simulink model "Robot_Control"  (Simulink 7.7)
settings: Solver=ode1  StartTime=0.0  StopTime=inf  FixedStep=0.002  RelTol=1e-3
values from neighbouring files (symbols this model uses):
  k = place(A,B,p)    [BalancePoles.m]
undefined symbols (not defined in the file or in its folder): HIL
libraries: quarc_library x4, simulink x1
settings Model: Creator=rcb4  LastModifiedBy=rcb4  SimulationMode=external  ExtModeTrigDuration=5000
settings SolverCC: PositivePriorityOrder=on
settings RTWCC: SystemTargetFile=quarc_win64.tlc  TemplateMakefile=quarc_default_tmf  Description=QUARC Win64 Target  ProcessScript=quarc_win64_make_rtw_hook
settings STFCustomTargetCC: TargetPreCompLibLocation=C:\PROGRA~3\QUARC\lib\2011a\win64\release  FunctionExecutionProfile=off  GeneratePreprocessorConditionals=Disable all  SystemTargetFile=quarc_win64.tlc
settings GRTTargetCC: TargetPreCompLibLocation=C:\PROGRA~3\QUARC\lib\2011a\win64\release  ParMdlRefBuildCompliant=off  CompOptLevelCompliant=off  MatFileLogging=off  ExtMode=on  ExtModeMexFile=quarc_comm

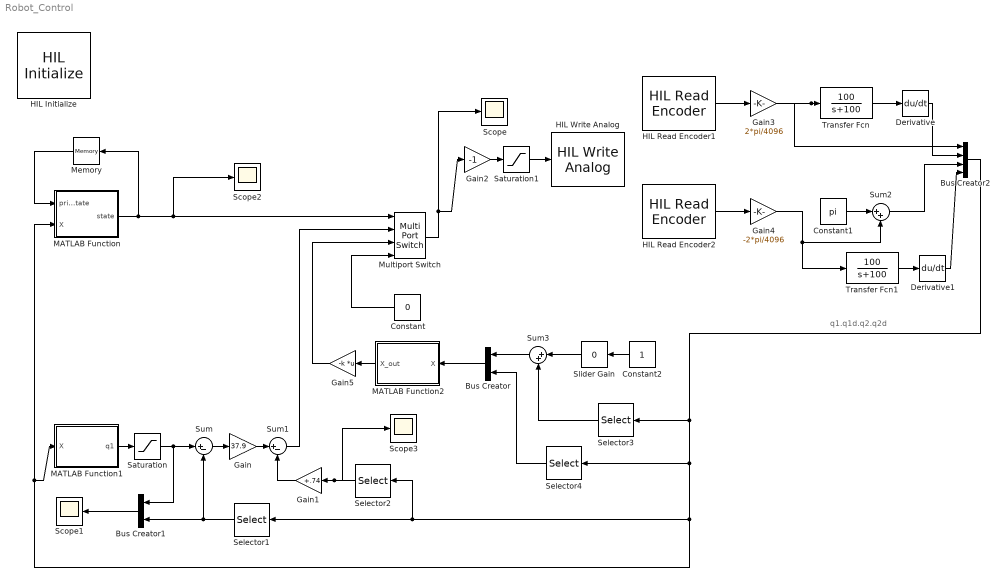
== system Robot_Control ==
  note: q1.q1d.q2.q2d
  Bus Creator : BusCreator  Inputs=2
  Bus Creator1 : BusCreator  Inputs=2
  Bus Creator2 : BusCreator
  Constant : Constant  Value=0
  Constant1 : Constant  Value=pi
  Constant2 : Constant
  Derivative : Derivative
  Derivative1 : Derivative
  Gain : Gain  Gain=37.9
  Gain1 : Gain  Gain=+.74
  Gain2 : Gain  Gain=-1
  Gain3 : Gain  Gain=2*pi/4096
  Gain4 : Gain  Gain=-2*pi/4096
  Gain5 : Gain  Gain=-k  Multiplication=Matrix(K*u)
  HIL Initialize : quarc_library/Data Acquisition/Generic/Configuration/HIL Initialize  object_name=HIL-1  board_type=q2_usb  board_number=0  board_options=d0=digital;d1=digital;led=auto;update_rate=normal;decimation=1  exclusive=off  active=off  hardware_clocks=[0:2]  clock_modes=[]  initial_clock_frequencies=[]  set_clock_params_at_start=off  set_clock_params_at_switch_in=off  set_clock_frequencies_at_start=off  set_clock_frequencies_at_switch_in=off  analog_input_channels=[0:1]  analog_input_maximums=10  analog_input_minimums=-10  set_analog_input_params_at_start=on  set_analog_input_params_at_switch_in=off  analog_output_channels=[0:1]  analog_output_maximums=10  analog_output_minimums=-10  initial_analog_outputs=[0]  final_analog_outputs=[0]  watchdog_analog_outputs=0  set_analog_output_params_at_start=on  set_analog_output_params_at_switch_in=off  set_analog_outputs_at_start=on  set_analog_outputs_at_switch_in=off  set_analog_outputs_at_terminate=on  set_analog_outputs_at_switch_out=off  set_analog_outputs_on_watchdog=off  digital_input_channels=[]  digital_output_channels=[]  digital_output_configuration=[]  initial_digital_outputs=[1]  final_digital_outputs=[1]  watchdog_digital_outputs=[1]  set_digital_output_params_at_start=off  set_digital_output_params_at_switch_in=off  set_digital_outputs_at_start=on  set_digital_outputs_at_switch_in=off  set_digital_outputs_at_terminate=on  set_digital_outputs_at_switch_out=off  set_digital_outputs_on_watchdog=off  encoder_channels=[0:1]  quadrature=[4]  encoder_filter_frequency=[]  initial_encoder_counts=[0]  set_encoder_params_at_start=on  set_encoder_params_at_switch_in=off  set_encoder_counts_at_start=on  set_encoder_counts_at_switch_in=off  pwm_channels=[]  pwm_modes=[0]  pwm_frequency=1/0.020  pwm_configuration=[]  pwm_alignment=[]  pwm_polarity=[]  pwm_leading_deadband=[]  pwm_trailing_deadband=[]  initial_pwm_outputs=[0]  final_pwm_outputs=[0]  watchdog_pwm_outputs=[0]  set_pwm_params_at_start=on  set_pwm_params_at_switch_in=off  set_pwm_outputs_at_start=on  set_pwm_outputs_at_switch_in=off  set_pwm_outputs_at_terminate=on  set_pwm_outputs_at_switch_out=off  set_pwm_outputs_on_watchdog=off  other_output_channels=[]  initial_other_outputs=[]  final_other_outputs=[]  watchdog_other_outputs=[]  set_other_outputs_at_start=off  set_other_outputs_at_switch_in=off  set_other_outputs_at_terminate=off  set_other_outputs_at_switch_out=off  set_other_outputs_on_watchdog=off
  HIL Read Encoder1 : quarc_library/Data Acquisition/Generic/Immediate I//O/HIL Read Encoder  object_name=HIL-1  channels=0  sample_time=qc_get_step_size  active=on  vector_output=off  data_type_mode=Inherit via back propagation  data_type=double
  HIL Read Encoder2 : quarc_library/Data Acquisition/Generic/Immediate I//O/HIL Read Encoder  object_name=HIL-1  channels=1  sample_time=qc_get_step_size  active=on  vector_output=off  data_type_mode=Inherit via back propagation  data_type=double
  HIL Write Analog : quarc_library/Data Acquisition/Generic/Immediate I//O/HIL Write Analog  object_name=HIL-1  channels=0  sample_time=-1  active=off  vector_input=off
  MATLAB Function : Stateflow chart  TreatAsAtomicUnit=on
  MATLAB Function1 : Stateflow chart  TreatAsAtomicUnit=on
  MATLAB Function2 : Stateflow chart  TreatAsAtomicUnit=on
  Memory : Memory
  Multiport Switch : MultiPortSwitch  DataPortOrder=Specify indices  DataPortIndices={0,1,2}  zeroidx=off
  Saturation : Saturate  UpperLimit=pi/2  LowerLimit=-pi/2
  Saturation1 : Saturate  UpperLimit=10  LowerLimit=-10
  Scope{,1..3} (4 alike) : Scope
      Scope settings: YMin=-0.05  YMax=0.8  DataFormat=Array
      Scope1 settings: YMin=-0.75  YMax=3
      Scope2 settings: YMin=-1  YMax=3  SaveName=ScopeData2
      Scope3 settings: YMin=-1  YMax=3  SaveName=ScopeData3
  Selector1 : Selector  InputPortWidth=4  IndexOptions=Index vector (dialog)  Indices=[1]  OutputSizes=1
  Selector2 : Selector  InputPortWidth=4  IndexOptions=Index vector (dialog)  Indices=[2]  OutputSizes=1
  Selector3 : Selector  InputPortWidth=4  IndexOptions=Index vector (dialog)  Indices=[1]  OutputSizes=1
  Selector4 : Selector  InputPortWidth=4  IndexOptions=Index vector (dialog)  Indices=[2,3,4]  OutputSizes=1
  Slider Gain : simulink/Math Operations/Slider Gain  SystemSampleTime=-1  low=-1.4  gain=0  high=1.4
  Sum : Sum  Inputs=|+-
  Sum1 : Sum  Inputs=|+-
  Sum2 : Sum  Inputs=|++
  Sum3 : Sum  Inputs=|++
  Transfer Fcn : TransferFcn  Numerator=[100]  Denominator=[1 100]
  Transfer Fcn1 : TransferFcn  Numerator=[100]  Denominator=[1 100]
  wires:
  MATLAB Function1/1(q1) -> Saturation/1
  MATLAB Function/1(state) -> Memory/1, Scope2/1, Multiport Switch/1
  Multiport Switch/1 -> Scope/1, Gain2/1
  Constant/1 -> Multiport Switch/4
  Sum1/1 -> Multiport Switch/2
  Gain/1 -> Sum1/1
  Gain1/1 -> Sum1/2
  Selector1/1 -> Sum/2, Bus Creator1/2
  Selector2/1 -> Gain1/1, Scope3/1
  Bus Creator1/1 -> Scope1/1
  Memory/1 -> MATLAB Function/1(prior_state)
  Sum/1 -> Gain/1
  Saturation/1 -> Bus Creator1/1, Sum/1
  HIL Read Encoder1/1 -> Gain3/1
  Bus Creator2/1 -> Selector3/1, MATLAB Function/2(X), MATLAB Function1/1(X), Selector1/1, Selector2/1, Selector4/1
  Gain3/1 -> Transfer Fcn/1, Bus Creator2/1
  Gain4/1 -> Transfer Fcn1/1, Sum2/2
  Transfer Fcn/1 -> Derivative/1
  Derivative/1 -> Bus Creator2/2
  Transfer Fcn1/1 -> Derivative1/1
  Constant1/1 -> Sum2/1
  Sum2/1 -> Bus Creator2/3
  Gain2/1 -> Saturation1/1
  Saturation1/1 -> HIL Write Analog/1
  HIL Read Encoder2/1 -> Gain4/1
  Derivative1/1 -> Bus Creator2/4
  MATLAB Function2/1(X_out) -> Gain5/1
  Gain5/1 -> Multiport Switch/3
  Constant2/1 -> Slider Gain/1
  Slider Gain/1 -> Sum3/1
  Selector3/1 -> Sum3/2
  Selector4/1 -> Bus Creator/2
  Sum3/1 -> Bus Creator/1
  Bus Creator/1 -> MATLAB Function2/1(X)

== matlab function MATLAB Function1 ==
  data: X input double; q1 output double
function q1 = fcn(X)
%return q1 based on q2 and q2d

P = .7;
D = .1;

q2 = X(3)-3.1;
q2d = X(4);

q2 = atan2(sin(q2),cos(q2));

q1 = P*q2 + D* q2d;

== matlab function MATLAB Function ==
  data: prior_state input double; X input double; state output double
function state = fcn(prior_state, X)

%SWINGUP switch function to pick which controller the robot uses


q2 = X(3);%mod( X(3) + pi/2, pi) - pi/2
q2 = atan2(sin(q2),cos(q2));
q2d = X(4);

errorTop = pi/4;
errorBot = pi/8;
errord = .05;

% swing = 0, balance = 1, wait = 2

q2_close_to_bottom = abs(q2 - pi)<errorBot;
q2d_is_small = abs(q2d)<errord;
q2_close_to_top = abs(q2)<errorTop;

if q2_close_to_bottom && q2d_is_small
    state = 0; % swing
elseif q2_close_to_top 
    state = 1; % balance
elseif ~q2_close_to_top && (prior_state==1)
    state = 2; %wait
elseif (prior_state==2) && ( ~q2_close_to_bottom || ~q2d_is_small)
    state = 2; % wait
else
   state = 0; % swing
end

end

== matlab function MATLAB Function2 ==
  data: X input double; X_out output double
function X_out = fcn(X)

X_out=X;
X_out(1) = X_out(1);
X_out(3)=asin(sin(X(3)));
